simulink model "model"  (R2016a)
(part 3 of 3)

  T_169122898_500000_東部変電所/RConn1 -- L_169122898/LConn1
  T_169122898_500000_東部変電所/RConn2 -- L_169122898/LConn2
  T_169122898_500000_東部変電所/RConn3 -- L_169122898/LConn3
  T_170247312_500000_新三河/RConn1 -- L_170247312/LConn1
  T_170247312_500000_新三河/RConn2 -- L_170247312/LConn2
  T_170247312_500000_新三河/RConn3 -- L_170247312/LConn3
  T_142662111_500000_中部電力㈱豊根開閉所/RConn1 -- L_142662111/LConn1
  T_142662111_500000_中部電力㈱豊根開閉所/RConn2 -- L_142662111/LConn2
  T_142662111_500000_中部電力㈱豊根開閉所/RConn3 -- L_142662111/LConn3
  T_170366035_500000_/RConn1 -- L_170366035/LConn1
  T_170366035_500000_/RConn2 -- L_170366035/LConn2
  T_170366035_500000_/RConn3 -- L_170366035/LConn3
  T_170850727_500000_愛知変電所/RConn1 -- L_170850727/LConn1
  T_170850727_500000_愛知変電所/RConn2 -- L_170850727/LConn2
  T_170850727_500000_愛知変電所/RConn3 -- L_170850727/LConn3
  T_170366036_275000_東豊田変電所/RConn1 -- L_170366036/LConn1
  T_170366036_275000_東豊田変電所/RConn2 -- L_170366036/LConn2
  T_170366036_275000_東豊田変電所/RConn3 -- L_170366036/LConn3
  T_170247359_275000_/RConn1 -- L_170247359/LConn1
  T_170247359_275000_/RConn2 -- L_170247359/LConn2
  T_170247359_275000_/RConn3 -- L_170247359/LConn3
  T_170366038_275000_/RConn1 -- L_170366038/LConn1
  T_170366038_275000_/RConn2 -- L_170366038/LConn2
  T_170366038_275000_/RConn3 -- L_170366038/LConn3
  T_242103481_500000_日野変電所/RConn1 -- L_242103481/LConn1
  T_242103481_500000_日野変電所/RConn2 -- L_242103481/LConn2
  T_242103481_500000_日野変電所/RConn3 -- L_242103481/LConn3
  T_241828221_500000_新岡山変電所_(Shin_Okayama_Hendensho)/RConn1 -- L_241828221/LConn1
  T_241828221_500000_新岡山変電所_(Shin_Okayama_Hendensho)/RConn2 -- L_241828221/LConn2
  T_241828221_500000_新岡山変電所_(Shin_Okayama_Hendensho)/RConn3 -- L_241828221/LConn3
  T_317511904_500000_北松江変電所/RConn1 -- L_317511904/LConn1
  T_317511904_500000_北松江変電所/RConn2 -- L_317511904/LConn2
  T_317511904_500000_北松江変電所/RConn3 -- L_317511904/LConn3
  T_241956440_275000_伊勢開閉所/RConn1 -- L_241956440/LConn1
  T_241956440_275000_伊勢開閉所/RConn2 -- L_241956440/LConn2
  T_241956440_275000_伊勢開閉所/RConn3 -- L_241956440/LConn3
  T_242532736_275000_/RConn1 -- L_242532736/LConn1
  T_242532736_275000_/RConn2 -- L_242532736/LConn2
  T_242532736_275000_/RConn3 -- L_242532736/LConn3
  T_170793703_275000_西尾張/RConn1 -- L_170793703/LConn1
  T_170793703_275000_西尾張/RConn2 -- L_170793703/LConn2
  T_170793703_275000_西尾張/RConn3 -- L_170793703/LConn3
  T_241923317_275000_南勢変電所_(Nansei_Hendensho)/RConn1 -- L_241923317/LConn1
  T_241923317_275000_南勢変電所_(Nansei_Hendensho)/RConn2 -- L_241923317/LConn2
  T_241923317_275000_南勢変電所_(Nansei_Hendensho)/RConn3 -- L_241923317/LConn3
  T_87682157_275000_南川越変電所_(Minamikawagoe_Hendensho)/RConn1 -- L_87682157/LConn1
  T_87682157_275000_南川越変電所_(Minamikawagoe_Hendensho)/RConn2 -- L_87682157/LConn2
  T_87682157_275000_南川越変電所_(Minamikawagoe_Hendensho)/RConn3 -- L_87682157/LConn3
  T_159491797_275000_南狭山変電所_(Minamisayama_Hendensho)/RConn1 -- L_159491797/LConn1
  T_159491797_275000_南狭山変電所_(Minamisayama_Hendensho)/RConn2 -- L_159491797/LConn2
  T_159491797_275000_南狭山変電所_(Minamisayama_Hendensho)/RConn3 -- L_159491797/LConn3
  T_105291887_275000_那珂変電所_(Naka_Hendensho)/RConn1 -- L_105291887/LConn1
  T_105291887_275000_那珂変電所_(Naka_Hendensho)/RConn2 -- L_105291887/LConn2
  T_105291887_275000_那珂変電所_(Naka_Hendensho)/RConn3 -- L_105291887/LConn3
  T_320438391_500000_/RConn1 -- L_320438391/LConn1
  T_320438391_500000_/RConn2 -- L_320438391/LConn2
  T_320438391_500000_/RConn3 -- L_320438391/LConn3
  T_241822621_500000_/RConn1 -- L_241822621/LConn1
  T_241822621_500000_/RConn2 -- L_241822621/LConn2
  T_241822621_500000_/RConn3 -- L_241822621/LConn3
  T_110682956_500000_猪名川変電所/RConn1 -- L_110682956/LConn1
  T_110682956_500000_猪名川変電所/RConn2 -- L_110682956/LConn2
  T_110682956_500000_猪名川変電所/RConn3 -- L_110682956/LConn3
  T_320444665_500000_/RConn1 -- L_320444665/LConn1
  T_320444665_500000_/RConn2 -- L_320444665/LConn2
  T_320444665_500000_/RConn3 -- L_320444665/LConn3
  T_179417733_275000_/RConn1 -- L_179417733/LConn1
  T_179417733_275000_/RConn2 -- L_179417733/LConn2
  T_179417733_275000_/RConn3 -- L_179417733/LConn3
  T_315461259_500000_/RConn1 -- L_315461259/LConn1
  T_315461259_500000_/RConn2 -- L_315461259/LConn2
  T_315461259_500000_/RConn3 -- L_315461259/LConn3
  T_315461272_500000_新木更津変電所/RConn1 -- L_315461272/LConn1
  T_315461272_500000_新木更津変電所/RConn2 -- L_315461272/LConn2
  T_315461272_500000_新木更津変電所/RConn3 -- L_315461272/LConn3
  T_170247308_275000_三河変電所/RConn1 -- L_170247308/LConn1
  T_170247308_275000_三河変電所/RConn2 -- L_170247308/LConn2
  T_170247308_275000_三河変電所/RConn3 -- L_170247308/LConn3
  T_170260165_275000_中部電力湖西変電所/RConn1 -- L_170260165/LConn1
  T_170260165_275000_中部電力湖西変電所/RConn2 -- L_170260165/LConn2
  T_170260165_275000_中部電力湖西変電所/RConn3 -- L_170260165/LConn3
  T_133137636_275000_北東京変電所_(Kita_Tōkyō_Hendensho)/RConn1 -- L_133137636/LConn1
  T_133137636_275000_北東京変電所_(Kita_Tōkyō_Hendensho)/RConn2 -- L_133137636/LConn2
  T_133137636_275000_北東京変電所_(Kita_Tōkyō_Hendensho)/RConn3 -- L_133137636/LConn3
  T_133641619_500000_新所沢変電所_(Shin_Tokorozawa_Hendensho)/RConn1 -- L_133641619/LConn1
  T_133641619_500000_新所沢変電所_(Shin_Tokorozawa_Hendensho)/RConn2 -- L_133641619/LConn2
  T_133641619_500000_新所沢変電所_(Shin_Tokorozawa_Hendensho)/RConn3 -- L_133641619/LConn3
  T_170247314_275000_額田開閉所/RConn1 -- L_170247314/LConn1
  T_170247314_275000_額田開閉所/RConn2 -- L_170247314/LConn2
  T_170247314_275000_額田開閉所/RConn3 -- L_170247314/LConn3
  T_315608215_500000_/RConn1 -- L_315608215/LConn1
  T_315608215_500000_/RConn2 -- L_315608215/LConn2
  T_315608215_500000_/RConn3 -- L_315608215/LConn3
  T_169249243_500000_南福光変電所/RConn1 -- L_169249243/LConn1
  T_169249243_500000_南福光変電所/RConn2 -- L_169249243/LConn2
  T_169249243_500000_南福光変電所/RConn3 -- L_169249243/LConn3
  T_169249247_500000_加賀変電所/RConn1 -- L_169249247/LConn1
  T_169249247_500000_加賀変電所/RConn2 -- L_169249247/LConn2
  T_169249247_500000_加賀変電所/RConn3 -- L_169249247/LConn3
  T_105298089_500000_新佐原変電所/RConn1 -- L_105298089/LConn1
  T_105298089_500000_新佐原変電所/RConn2 -- L_105298089/LConn2
  T_105298089_500000_新佐原変電所/RConn3 -- L_105298089/LConn3
  T_153521822_275000_西越谷変電所_(Nishi_Koshigaya_Hendensho)/RConn1 -- L_153521822/LConn1
  T_153521822_275000_西越谷変電所_(Nishi_Koshigaya_Hendensho)/RConn2 -- L_153521822/LConn2
  T_153521822_275000_西越谷変電所_(Nishi_Koshigaya_Hendensho)/RConn3 -- L_153521822/LConn3
  T_204258596_500000_/RConn1 -- L_204258596/LConn1
  T_204258596_500000_/RConn2 -- L_204258596/LConn2
  T_204258596_500000_/RConn3 -- L_204258596/LConn3
  T_87538349_500000_讃岐変電所/RConn1 -- L_87538349/LConn1
  T_87538349_500000_讃岐変電所/RConn2 -- L_87538349/LConn2
  T_87538349_500000_讃岐変電所/RConn3 -- L_87538349/LConn3
  T_171066843_500000_四国電力東予変電所/RConn1 -- L_171066843/LConn1
  T_171066843_500000_四国電力東予変電所/RConn2 -- L_171066843/LConn2
  T_171066843_500000_四国電力東予変電所/RConn3 -- L_171066843/LConn3
  T_102958903_500000_/RConn1 -- L_102958903/LConn1
  T_102958903_500000_/RConn2 -- L_102958903/LConn2
  T_102958903_500000_/RConn3 -- L_102958903/LConn3
  T_242253497_275000_姫路変電所_(Himeji_Hendensho)/RConn1 -- L_242253497/LConn1
  T_242253497_275000_姫路変電所_(Himeji_Hendensho)/RConn2 -- L_242253497/LConn2
  T_242253497_275000_姫路変電所_(Himeji_Hendensho)/RConn3 -- L_242253497/LConn3
  T_185032690_275000_西神戸変電所/RConn1 -- L_185032690/LConn1
  T_185032690_275000_西神戸変電所/RConn2 -- L_185032690/LConn2
  T_185032690_275000_西神戸変電所/RConn3 -- L_185032690/LConn3
  T_160374974_275000;77000_北葛城変電所_(Kita_Katsuragi_Hendensho)/RConn1 -- L_160374974/LConn1
  T_160374974_275000;77000_北葛城変電所_(Kita_Katsuragi_Hendensho)/RConn2 -- L_160374974/LConn2
  T_160374974_275000;77000_北葛城変電所_(Kita_Katsuragi_Hendensho)/RConn3 -- L_160374974/LConn3
  T_302164679_275000_能代変電所/RConn1 -- L_302164679/LConn1
  T_302164679_275000_能代変電所/RConn2 -- L_302164679/LConn2
  T_302164679_275000_能代変電所/RConn3 -- L_302164679/LConn3
  T_316581637_275000_青森変電所/RConn1 -- L_316581637/LConn1
  T_316581637_275000_青森変電所/RConn2 -- L_316581637/LConn2
  T_316581637_275000_青森変電所/RConn3 -- L_316581637/LConn3
  T_216956620_500000_/RConn1 -- L_216956620/LConn1
  T_216956620_500000_/RConn2 -- L_216956620/LConn2
  T_216956620_500000_/RConn3 -- L_216956620/LConn3
  T_159191758_275000_北松本変電所/RConn1 -- L_159191758/LConn1
  T_159191758_275000_北松本変電所/RConn2 -- L_159191758/LConn2
  T_159191758_275000_北松本変電所/RConn3 -- L_159191758/LConn3
  T_211258348_275000_東信変電所/RConn1 -- L_211258348/LConn1
  T_211258348_275000_東信変電所/RConn2 -- L_211258348/LConn2
  T_211258348_275000_東信変電所/RConn3 -- L_211258348/LConn3
  T_169963227_500000_新榛名/RConn1 -- L_169963227/LConn1
  T_169963227_500000_新榛名/RConn2 -- L_169963227/LConn2
  T_169963227_500000_新榛名/RConn3 -- L_169963227/LConn3
  T_195615141_500000_/RConn1 -- L_195615141/LConn1
  T_195615141_500000_/RConn2 -- L_195615141/LConn2
  T_195615141_500000_/RConn3 -- L_195615141/LConn3
  T_199544541_275000_新北信変電所/RConn1 -- L_199544541/LConn1
  T_199544541_275000_新北信変電所/RConn2 -- L_199544541/LConn2
  T_199544541_275000_新北信変電所/RConn3 -- L_199544541/LConn3
  T_190734269_275000_/RConn1 -- L_190734269/LConn1
  T_190734269_275000_/RConn2 -- L_190734269/LConn2
  T_190734269_275000_/RConn3 -- L_190734269/LConn3
  T_161948515_275000_西濃変電所_(Seinō_Hendensho)/RConn1 -- L_161948515/LConn1
  T_161948515_275000_西濃変電所_(Seinō_Hendensho)/RConn2 -- L_161948515/LConn2
  T_161948515_275000_西濃変電所_(Seinō_Hendensho)/RConn3 -- L_161948515/LConn3
  T_170793702_275000_西名古屋/RConn1 -- L_170793702/LConn1
  T_170793702_275000_西名古屋/RConn2 -- L_170793702/LConn2
  T_170793702_275000_西名古屋/RConn3 -- L_170793702/LConn3
  T_242103532_500000_/RConn1 -- L_242103532/LConn1
  T_242103532_500000_/RConn2 -- L_242103532/LConn2
  T_242103532_500000_/RConn3 -- L_242103532/LConn3
  T_241822623_500000;220000;110000_/RConn1 -- L_241822623/LConn1
  T_241822623_500000;220000;110000_/RConn2 -- L_241822623/LConn2
  T_241822623_500000;220000;110000_/RConn3 -- L_241822623/LConn3
  T_47110637_275000_西東京変電所/RConn1 -- L_47110637/LConn1
  T_47110637_275000_西東京変電所/RConn2 -- L_47110637/LConn2
  T_47110637_275000_西東京変電所/RConn3 -- L_47110637/LConn3
  T_104375141_275000_須賀川変電所_(Sukagawa_Hendensho)/RConn1 -- L_104375141/LConn1
  T_104375141_275000_須賀川変電所_(Sukagawa_Hendensho)/RConn2 -- L_104375141/LConn2
  T_104375141_275000_須賀川変電所_(Sukagawa_Hendensho)/RConn3 -- L_104375141/LConn3
  T_107262429_275000_福島変電所/RConn1 -- L_107262429/LConn1
  T_107262429_275000_福島変電所/RConn2 -- L_107262429/LConn2
  T_107262429_275000_福島変電所/RConn3 -- L_107262429/LConn3
  T_250540807_500000_東群馬変電所_(Higashi_Gunma_Substation)/RConn1 -- L_250540807/LConn1
  T_250540807_500000_東群馬変電所_(Higashi_Gunma_Substation)/RConn2 -- L_250540807/LConn2
  T_250540807_500000_東群馬変電所_(Higashi_Gunma_Substation)/RConn3 -- L_250540807/LConn3
  T_291678103_275000_紀の川変電所_(Kinokawa_Hendensho)/RConn1 -- L_291678103/LConn1
  T_291678103_275000_紀の川変電所_(Kinokawa_Hendensho)/RConn2 -- L_291678103/LConn2
  T_291678103_275000_紀の川変電所_(Kinokawa_Hendensho)/RConn3 -- L_291678103/LConn3
  T_151379730_500000_房総変電所_(Bōsō_Hendensho)/RConn1 -- L_151379730/LConn1
  T_151379730_500000_房総変電所_(Bōsō_Hendensho)/RConn2 -- L_151379730/LConn2
  T_151379730_500000_房総変電所_(Bōsō_Hendensho)/RConn3 -- L_151379730/LConn3
  T_168727982_500000_新京葉変電所/RConn1 -- L_168727982/LConn1
  T_168727982_500000_新京葉変電所/RConn2 -- L_168727982/LConn2
  T_168727982_500000_新京葉変電所/RConn3 -- L_168727982/LConn3
  T_215451416_500000;220000_九州電力南九州変電所/RConn1 -- L_215451416/LConn1
  T_215451416_500000;220000_九州電力南九州変電所/RConn2 -- L_215451416/LConn2
  T_215451416_500000;220000_九州電力南九州変電所/RConn3 -- L_215451416/LConn3
  T_325868333_275000_/RConn1 -- L_325868333/LConn1
  T_325868333_275000_/RConn2 -- L_325868333/LConn2
  T_325868333_275000_/RConn3 -- L_325868333/LConn3
  T_110682951_275000_宝塚開閉所_(Takarazuka_Kaiheisho)/RConn1 -- L_110682951/LConn1
  T_110682951_275000_宝塚開閉所_(Takarazuka_Kaiheisho)/RConn2 -- L_110682951/LConn2
  T_110682951_275000_宝塚開閉所_(Takarazuka_Kaiheisho)/RConn3 -- L_110682951/LConn3
  T_145080115_275000_/RConn1 -- L_145080115/LConn1
  T_145080115_275000_/RConn2 -- L_145080115/LConn2
  T_145080115_275000_/RConn3 -- L_145080115/LConn3
  T_133135172_500000_新古河変電所/RConn1 -- L_133135172/LConn1
  T_133135172_500000_新古河変電所/RConn2 -- L_133135172/LConn2
  T_133135172_500000_新古河変電所/RConn3 -- L_133135172/LConn3
  T_132913106_500000_新筑波変電所_(Shin_Tsukuba_Hendensho)/RConn1 -- L_132913106/LConn1
  T_132913106_500000_新筑波変電所_(Shin_Tsukuba_Hendensho)/RConn2 -- L_132913106/LConn2
  T_132913106_500000_新筑波変電所_(Shin_Tsukuba_Hendensho)/RConn3 -- L_132913106/LConn3
  T_110682955_275000;154000;77000_伊丹変電所_(Itami_Hendensho)/RConn1 -- L_110682955/LConn1
  T_110682955_275000;154000;77000_伊丹変電所_(Itami_Hendensho)/RConn2 -- L_110682955/LConn2
  T_110682955_275000;154000;77000_伊丹変電所_(Itami_Hendensho)/RConn3 -- L_110682955/LConn3
  T_318302348_275000_東上越変電所/RConn1 -- L_318302348/LConn1
  T_318302348_275000_東上越変電所/RConn2 -- L_318302348/LConn2
  T_318302348_275000_東上越変電所/RConn3 -- L_318302348/LConn3
  T_170605907_500000_北摂変電所/RConn1 -- L_170605907/LConn1
  T_170605907_500000_北摂変電所/RConn2 -- L_170605907/LConn2
  T_170605907_500000_北摂変電所/RConn3 -- L_170605907/LConn3
  T_185029969_500000;220000_/RConn1 -- L_185029969/LConn1
  T_185029969_500000;220000_/RConn2 -- L_185029969/LConn2
  T_185029969_500000;220000_/RConn3 -- L_185029969/LConn3
  T_316459359_275000_/RConn1 -- L_316459359/LConn1
  T_316459359_275000_/RConn2 -- L_316459359/LConn2
  T_316459359_275000_/RConn3 -- L_316459359/LConn3
  T_104391636_500000_新いわき/RConn1 -- L_104391636/LConn1
  T_104391636_500000_新いわき/RConn2 -- L_104391636/LConn2
  T_104391636_500000_新いわき/RConn3 -- L_104391636/LConn3
  T_190984572_275000_/RConn1 -- L_190984572/LConn1
  T_190984572_275000_/RConn2 -- L_190984572/LConn2
  T_190984572_275000_/RConn3 -- L_190984572/LConn3
  T_209726348_500000_信濃変電所/RConn1 -- L_209726348/LConn1
  T_209726348_500000_信濃変電所/RConn2 -- L_209726348/LConn2
  T_209726348_500000_信濃変電所/RConn3 -- L_209726348/LConn3
  T_209429410_500000_南信変電所/RConn1 -- L_209429410/LConn1
  T_209429410_500000_南信変電所/RConn2 -- L_209429410/LConn2
  T_209429410_500000_南信変電所/RConn3 -- L_209429410/LConn3
  T_315662839_500000_新信濃変電所/RConn1 -- L_315662839/LConn1
  T_315662839_500000_新信濃変電所/RConn2 -- L_315662839/LConn2
  T_315662839_500000_新信濃変電所/RConn3 -- L_315662839/LConn3
  T_109850439_500000_/RConn1 -- L_109850439/LConn1
  T_109850439_500000_/RConn2 -- L_109850439/LConn2
  T_109850439_500000_/RConn3 -- L_109850439/LConn3
